simulink model "discrete_four_chan_local_feedback"  (R2020b)
settings: Solver=ode45  StartTime=0.0  StopTime=5  RelTol=1e-3
values from neighbouring files (symbols this model uses):
  A = 1    [hw3_main.m]
  Be = 30    [hw3_main.m]
  Bh = 70    [hw3_main.m]
  Bm = 0.8    [hw3_main.m]
  Bs = 3.2    [hw3_main.m]
  Cmf = 0    [hw3_main.m]
  Csf = 0    [hw3_main.m]
  Dh = 1000    [hw3_main.m]
  Dm = 5    [hw3_main.m]
  Ds = 10    [hw3_main.m]
  Fc = 1    [hw3_main.m]
  Fip = 1    [hw3_main.m]
  Je = 0    [hw3_main.m]
  Jh = 0.5    [hw3_main.m]
  Ke = 50    [hw3_main.m]
  Kh = 2000    [hw3_main.m]
  Km = 1    [hw3_main.m]
  Ks = 4    [hw3_main.m]
  Mm = 0.5    [hw3_main.m]
  Ms = 2    [hw3_main.m]
  Ph = 20000    [hw3_main.m]
  posNoiseVar = 0.00001    (= 1e-05)    [hw3_main.m]
  torqueNoiseVar = 0.01    [hw3_main.m]
  Ts = 0.001    [hw3_main.m]
  xe = 2    [hw3_main.m]
libraries: simulink x4
settings Model: Creator=nicol  LastModifiedBy=nicol

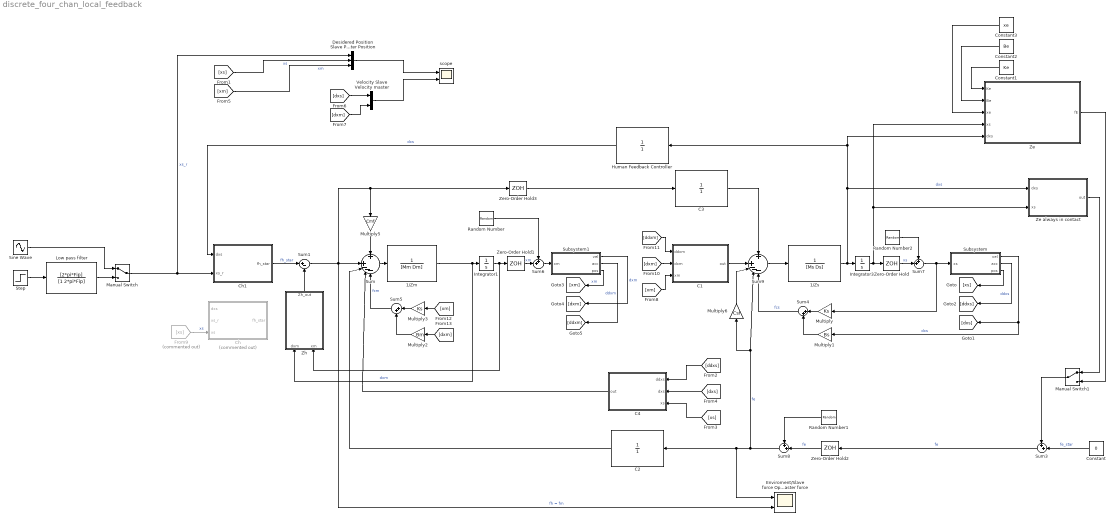
== system discrete_four_chan_local_feedback ==
  1/Zm : TransferFcn  Denominator=[Mm Dm]
  1/Zs : TransferFcn  Denominator=[Ms Ds]
  C1 : Subsystem
  C2 : TransferFcn  Denominator=[1]
  C3 : TransferFcn  Denominator=[1]
  C4 : Subsystem
  Ch : Subsystem  Commented=on
  Ch1 : Subsystem
  Constant : Constant  Value=0
  Constant1 : Constant  Value=Ke
  Constant2 : Constant  Value=Be
  Constant3 : Constant  Value=xe
  Desidered Position Slave Position Master Position : Mux  Inputs=3
  Enviroment/Slave force Operator/Master force : Scope  NumInputPorts=2
  From9 : From  Commented=on  GotoTag=xs
  Human Feedback Controller : TransferFcn  Denominator=[1]
  Integrator1 : Integrator
  Integrator3 : Integrator
  Low pass filter : TransferFcn  Numerator=[2*pi*Fip]  Denominator=[1 2*pi*Fip]
  Manual Switch : ManualSwitch
  Manual Switch1 : ManualSwitch
  Multiply : Gain  Gain=Ks
  Multiply1 : Gain  Gain=Bs
  Multiply2 : Gain  Gain=Bm
  Multiply3 : Gain  Gain=Ks
  Multiply5 : Gain  Gain=Cmf
  Multiply6 : Gain  Gain=Csf
  Random Number : RandomNumber  Variance=posNoiseVar  SampleTime=Ts
  Random Number1 : RandomNumber  Variance=torqueNoiseVar  SampleTime=Ts
  Random Number2 : RandomNumber  Variance=posNoiseVar  SampleTime=Ts
  Sine Wave : Sin  Amplitude=A  Frequency=2*pi*Fc  SampleTime=0
  Step : Step  After=A  SampleTime=0
  Subsystem : Subsystem
  Subsystem1 : Subsystem
  Sum : Sum  Inputs=+||+---
  Sum1 : Sum  Inputs=|+-
  Sum{3,6..8} (4 alike) : Sum  Inputs=++|
  Sum4 : Sum  Inputs=|++
  Sum5 : Sum  Inputs=|++
  Sum9 : Sum  Inputs=+||+---
  Velocity Slave Velocity master : Mux  Inputs=2
  Ze : MATLAB Function  TreatAsAtomicUnit=on
  Ze always in contact : Subsystem
  Zero-Order Hold{,1..3} (4 alike) : ZeroOrderHold  SampleTime=Ts
  Zh : Subsystem
  "scope " : Scope  NumInputPorts=2
  wires:
  Sine Wave/1 -> Manual Switch/1
  Zh/1(Zh_out) -> Sum1/2
  Subsystem1/1(vel) -> [dxm]  "dxm"
  Sum5/1 -> Sum/5  "fcm"
  Sum1/1 -> Multiply5/1, Zero-Order Hold3/1, Sum/2, Enviroment/Slave force Operator/Master force/2  "fh = fm"
  C2/1 -> Sum/3
  C4/1(out) -> Sum/4
  C1/1(out) -> Sum9/2
  C3/1 -> Sum9/1
  Sum4/1 -> Sum9/5  "fcs"
  Sum9/1 -> 1/Zs/1
  Ze/1(fE) -> Manual Switch1/2
  Sum3/1 -> Zero-Order Hold2/1  "fe"
  Human Feedback Controller/1 -> Ch1/1(dxs)  "dxs"
  Constant/1 -> Sum3/2  "fe_star"
  Constant1/1 -> Ze/1(Ke)
  Constant2/1 -> Ze/2(Be)
  Constant3/1 -> Ze/3(xe)
  Step/1 -> Low pass filter/1
  Manual Switch/1 -> Desidered Position Slave Position Master Position/1, Ch1/2(xs_r)  "xs_r"
  Low pass filter/1 -> Manual Switch/2
  Manual Switch1/1 -> Sum3/1
  Ze always in contact/1(out) -> Manual Switch1/1
  Sum/1 -> 1/Zm/1
  [xs] -> Desidered Position Slave Position Master Position/2  "xs"
  [xm] -> Desidered Position Slave Position Master Position/3  "xm"
  Velocity Slave Velocity master/1 -> "scope "/2
  Desidered Position Slave Position Master Position/1 -> "scope "/1
  1/Zs/1 -> Human Feedback Controller/1, Ze/5(dxs), Ze always in contact/1(dxs), Integrator3/1  "dxs"
  Subsystem/1(vel) -> [dxs], Multiply1/1  "dxs"
  Multiply/1 -> Sum4/1
  Multiply1/1 -> Sum4/2
  Integrator3/1 -> Ze/4(xs), Ze always in contact/2(xs), Zero-Order Hold/1
  Subsystem/2(acc) -> [ddxs]  "ddxs"
  [ddxs] -> C4/1(ddxs)
  [dxs] -> C4/2(dxs)
  [xs] -> C4/3(xs)
  Integrator1/1 -> Zh/2(xm), Zero-Order Hold1/1
  1/Zm/1 -> Integrator1/1, Zh/1(dxm)  "dxm"
  Subsystem1/2(acc) -> [ddxm]  "ddxm"
  Multiply3/1 -> Sum5/1
  Multiply2/1 -> Sum5/2
  [dxs] -> Velocity Slave Velocity master/1
  [dxm] -> Velocity Slave Velocity master/2
  [xm] -> C1/3(xm)
  Sum8/1 -> Enviroment/Slave force Operator/Master force/1, C2/1, Sum9/4, Multiply6/1  "fe"
  Zero-Order Hold3/1 -> C3/1
  Sum6/1 -> Subsystem1/1(xm)
  Random Number/1 -> Sum6/1
  Sum7/1 -> Multiply/1, Subsystem/1(xs)
  Random Number2/1 -> Sum7/1
  Zero-Order Hold1/1 -> Sum6/2  "xm"
  Zero-Order Hold/1 -> Sum7/2  "xs"
  Subsystem/3(pos) -> [xs]
  Subsystem1/3(pos) -> [xm]  "xm"
  [dxm] -> C1/2(dxm)
  [ddxm] -> C1/1(ddxm)
  Ch1/1(fh_star) -> Sum1/1  "fh_star"
  From9/1 -> Ch/3(xs)  "xs"
  Random Number1/1 -> Sum8/1
  Zero-Order Hold2/1 -> Sum8/2  "fe"
  [xm] -> Multiply3/1
  [dxm] -> Multiply2/1
  Multiply6/1 -> Sum9/3
  Multiply5/1 -> Sum/1

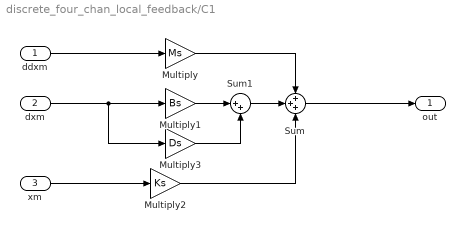
== system discrete_four_chan_local_feedback/C1 ==
  ddxm : Inport
  dxm : Inport  Port=2
  xm : Inport  Port=3
  Multiply : Gain  Gain=Ms
  Multiply1 : Gain  Gain=Bs
  Multiply2 : Gain  Gain=Ks
  Multiply3 : Gain  Gain=Ds
  Sum : Sum  Inputs=+++
  Sum1 : Sum  Inputs=|++
  out : Outport
  wires:
  ddxm/1 -> Multiply/1
  Sum/1 -> out/1
  xm/1 -> Multiply2/1
  Multiply1/1 -> Sum1/1
  Multiply/1 -> Sum/1
  Multiply2/1 -> Sum/3
  Sum1/1 -> Sum/2
  Multiply3/1 -> Sum1/2
  dxm/1 -> Multiply3/1, Multiply1/1

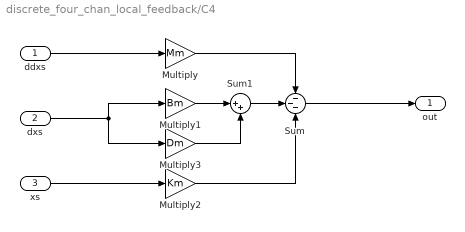
== system discrete_four_chan_local_feedback/C4 ==
  ddxs : Inport
  dxs : Inport  Port=2
  xs : Inport  Port=3
  Multiply : Gain  Gain=Mm
  Multiply1 : Gain  Gain=Bm
  Multiply2 : Gain  Gain=Km
  Multiply3 : Gain  Gain=Dm
  Sum : Sum  Inputs=---
  Sum1 : Sum  Inputs=|++
  out : Outport
  wires:
  ddxs/1 -> Multiply/1
  Sum/1 -> out/1
  xs/1 -> Multiply2/1
  Multiply1/1 -> Sum1/1
  Multiply/1 -> Sum/1
  Multiply2/1 -> Sum/3
  Sum1/1 -> Sum/2
  Multiply3/1 -> Sum1/2
  dxs/1 -> Multiply3/1, Multiply1/1

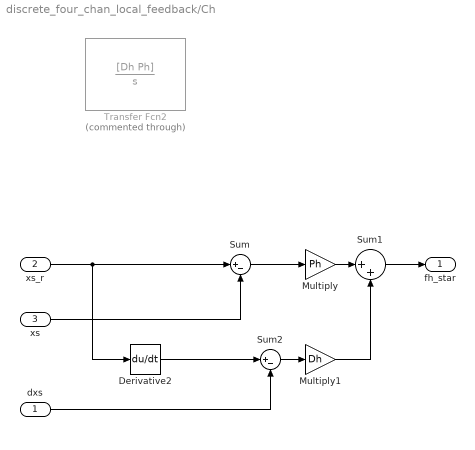
== system discrete_four_chan_local_feedback/Ch ==
  dxs : Inport
  xs_r : Inport  Port=2
  xs : Inport  Port=3
  Derivative2 : Derivative
  Multiply : Gain  Gain=Ph
  Multiply1 : Gain  Gain=Dh
  Sum : Sum  Inputs=|+-
  Sum1 : Sum  Inputs=|++
  Sum2 : Sum  Inputs=|+-
  Transfer Fcn2 : TransferFcn  Commented=through  Numerator=[Dh Ph]  Denominator=[1 0]
  fh_star : Outport
  wires:
  dxs/1 -> Sum2/2
  Sum/1 -> Multiply/1
  Sum1/1 -> fh_star/1
  xs_r/1 -> Derivative2/1, Sum/1
  xs/1 -> Sum/2
  Multiply/1 -> Sum1/1
  Multiply1/1 -> Sum1/2
  Derivative2/1 -> Sum2/1
  Sum2/1 -> Multiply1/1

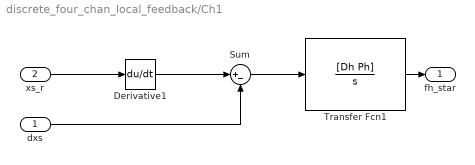
== system discrete_four_chan_local_feedback/Ch1 ==
  dxs : Inport
  xs_r : Inport  Port=2
  Derivative1 : Derivative
  Sum : Sum  Inputs=|+-
  Transfer Fcn1 : TransferFcn  Numerator=[Dh Ph]  Denominator=[1 0]
  fh_star : Outport
  wires:
  dxs/1 -> Sum/2
  Sum/1 -> Transfer Fcn1/1
  Transfer Fcn1/1 -> fh_star/1
  xs_r/1 -> Derivative1/1
  Derivative1/1 -> Sum/1

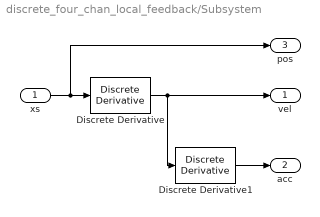
== system discrete_four_chan_local_feedback/Subsystem ==
  xs : Inport
  Discrete Derivative : simulink/Discrete/Discrete Derivative  gainval=1.0  ICPrevScaledInput=0.0  OutMin=[]  OutMax=[]  OutDataType=fixdt(1, 16)  OutScaling=2^-10  DoSatur=off
  Discrete Derivative1 : simulink/Discrete/Discrete Derivative  gainval=1.0  ICPrevScaledInput=0.0  OutMin=[]  OutMax=[]  OutDataType=fixdt(1, 16)  OutScaling=2^-10  DoSatur=off
  vel : Outport
  acc : Outport  Port=2
  pos : Outport  Port=3
  wires:
  xs/1 -> pos/1, Discrete Derivative/1
  Discrete Derivative/1 -> Discrete Derivative1/1, vel/1
  Discrete Derivative1/1 -> acc/1

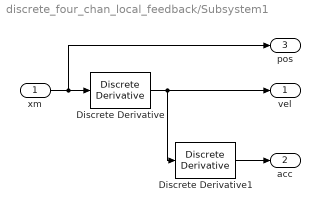
== system discrete_four_chan_local_feedback/Subsystem1 ==
  xm : Inport
  Discrete Derivative : simulink/Discrete/Discrete Derivative  gainval=1.0  ICPrevScaledInput=0.0  OutMin=[]  OutMax=[]  OutDataType=fixdt(1, 16)  OutScaling=2^-10  DoSatur=off
  Discrete Derivative1 : simulink/Discrete/Discrete Derivative  gainval=1.0  ICPrevScaledInput=0.0  OutMin=[]  OutMax=[]  OutDataType=fixdt(1, 16)  OutScaling=2^-10  DoSatur=off
  vel : Outport
  acc : Outport  Port=2
  pos : Outport  Port=3
  wires:
  xm/1 -> pos/1, Discrete Derivative/1
  Discrete Derivative/1 -> Discrete Derivative1/1, vel/1
  Discrete Derivative1/1 -> acc/1

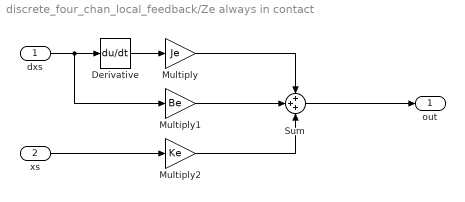
== system discrete_four_chan_local_feedback/Ze always in contact ==
  dxs : Inport
  xs : Inport  Port=2
  Derivative : Derivative
  Multiply : Gain  Gain=Je
  Multiply1 : Gain  Gain=Be
  Multiply2 : Gain  Gain=Ke
  Sum : Sum  Inputs=+++
  out : Outport
  wires:
  dxs/1 -> Multiply1/1, Derivative/1
  Derivative/1 -> Multiply/1
  Sum/1 -> out/1
  xs/1 -> Multiply2/1
  Multiply1/1 -> Sum/2
  Multiply/1 -> Sum/1
  Multiply2/1 -> Sum/3

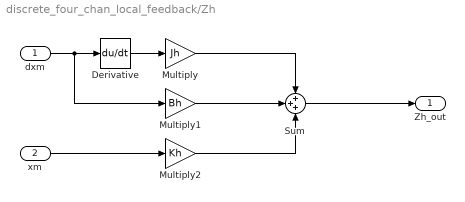
== system discrete_four_chan_local_feedback/Zh ==
  dxm : Inport
  xm : Inport  Port=2
  Derivative : Derivative
  Multiply : Gain  Gain=Jh
  Multiply1 : Gain  Gain=Bh
  Multiply2 : Gain  Gain=Kh
  Sum : Sum  Inputs=+++
  Zh_out : Outport
  wires:
  dxm/1 -> Multiply1/1, Derivative/1
  Derivative/1 -> Multiply/1
  Sum/1 -> Zh_out/1
  xm/1 -> Multiply2/1
  Multiply1/1 -> Sum/2
  Multiply/1 -> Sum/1
  Multiply2/1 -> Sum/3

== matlab function discrete_four_chan_local_feedback/Ze ==
  data: Ke input; fE output; Be input; xe input; xs input; dxs input
function fE = environment(Ke,Be,xe,xs,dxs)
if(xs>xe)
    fE=Ke*(xs-xe)+Be*dxs;
else
    fE=0;
end
